simulink model "phi2_m1_vr01_k2_2"  (R2024b)
settings: Solver=FixedStepAuto  StartTime=0.0  StopTime=24.0  FixedStep=1.0  RelTol=1e-3
libraries: deeplib x1
settings Model: Creator=ldy  LastModifiedBy=fedformi_new
settings DataIOCC: SaveFormat=Array  SignalLogging=off  DSMLogging=off

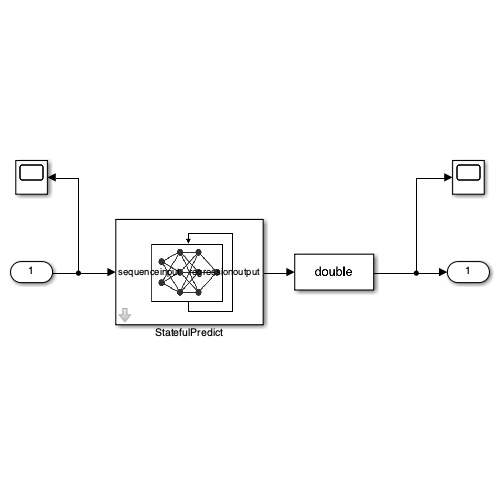
[thumbnail: Simulink's stored preview of the top-level diagram]
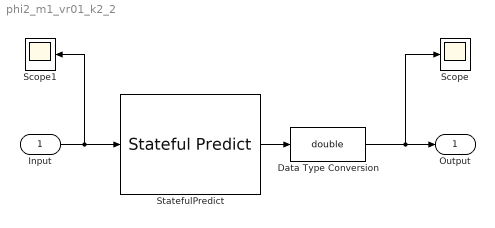
== system phi2_m1_vr01_k2_2 ==
  Input : Inport
  Data Type Conversion : DataTypeConversion  OutDataTypeStr=double  SaturateOnIntegerOverflow=off  RndMeth=Floor
  Scope : Scope
  Scope1 : Scope
  StatefulPredict : deeplib/Stateful Predict  Network=Network from MAT-file  NetworkFunction=untitled  NetworkFilePath=SB2-Synthetic_Benchmark_2/phi2_m1_vr01_k2_2.mat  InputDataFormats={'',''}  SampleTime=1  ForceInterpretedSim=off  EnableDLNetwork=on  LastKnownNetworkFilePath=''  LastKnownNetworkTimeStamp=''
  Output : Outport
  wires:
  Input/1 -> Scope1/1, StatefulPredict/1
  StatefulPredict/1 -> Data Type Conversion/1
  Data Type Conversion/1 -> Scope/1, Output/1
